simulink model "gcc"  (R2020a)
settings: Solver=ode23t  StartTime=0.0  StopTime=0.5  FixedStep=1e-6  RelTol=1e-3
undefined symbols (not defined in the file or in its folder): Ion, Lithium
libraries: powerlib x20, powerlib_extras x7, simulink x4, powerlib_meascontrol x2, electricdrivelib x1, re_lib x1
settings Model: Creator=kc  LastModifiedBy=BJ137
settings DataIOCC: SaveOutput=off  SignalLogging=off  DSMLogging=off  SaveTime=off  ReturnWorkspaceOutputs=off
settings OptimizationCC: LifeSpan=inf
settings DebuggingCC: ArithmeticOperatorsInVariantConditions=warning
settings SFSimCC: CustomCodeUndefinedFunction=UseInterfaceOnly
settings CodeAppCC: StateflowObjectComments=on

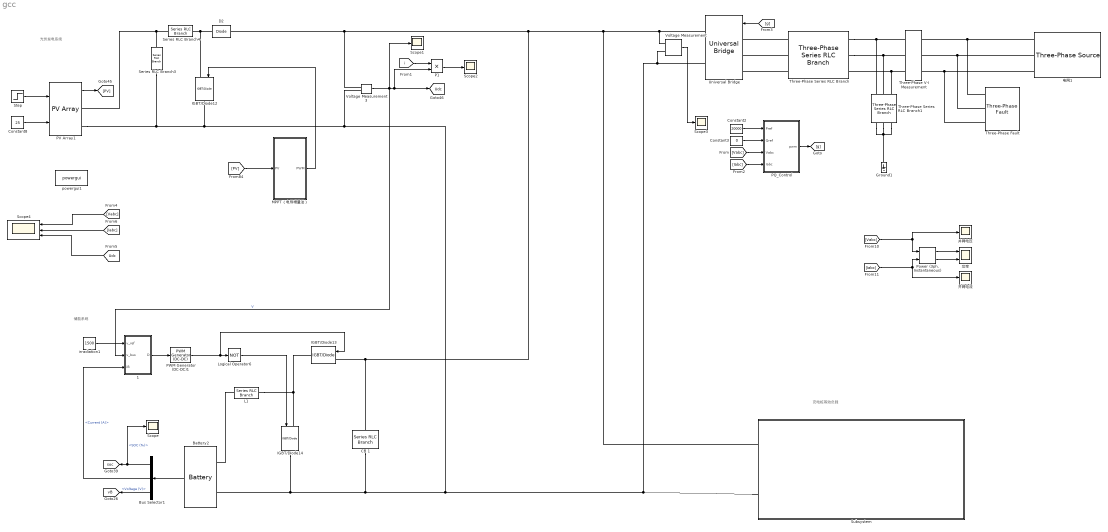
== system gcc ==
  note: 光伏发电系统
  note: 储能系统
  note: 充电桩等效负载
  1 : Subsystem
  Battery2 : electricdrivelib/Extra Sources/Battery  BatType=Lithium-Ion  ShowTempParam=off  ThermalPreset=no  ShowAgeParam=off  NomV=1000  NomQ=200  SOC=50  Batt_Tr=0  PresetModel=on  MaxQ=200  MinV=750  FullV=1163.9871  Dis_rate=86.9565  R=0.05  Normal_OP=180.8696  expZone="[1080.3859       9.826087]"  current=[6.5 13 32.5]  Units=Time  Tci=20  NomT=20  T2=-30  MaxQ2=4.8  FullV2=7.1  Normal_OP2=5.655  expZone2="[6.58           1]"  Rca=0.6  ti=2000  Dp=0  Neq0=0  Tsim=1e6  Ta1=25  Qeol=5.4*0.9  Reol=0.013333*1.2  Char_age=[2.3478, 3]  Dis_age=[2.3478, 10]  N1=1500  N2=10500  N3=1000  N4=1400  Ta2=45  N5=950
  Bus Selector1 : BusSelector  OutputSignals=SOC (%),Current (A),Voltage (V)
  CB 1 : powerlib/Elements/Series RLC Branch  LConnTagsString=__new0  RConnTagsString=__new0  BranchType=C  Resistance=1e-4  Inductance=1e-3  SetiL0=off  InitialCurrent=0  Capacitance=1000e-6  Setx0=on  InitialVoltage=800  Measurements=None
  Constant2 : Constant  Value=20000
  Constant3 : Constant  Value=0
  Constant8 : Constant  Value=25
  D2 : powerlib/Power Electronics/Diode  Ron=0.001  Lon=0  Vf=0  IC=0  UseSnubber=off  Rs=inf  Cs=inf  Measurements=off
  Ground1 : powerlib/Elements/Ground  LConnTagsString=a
  IGBT/Diode12 : powerlib/Power Electronics/IGBT//Diode  Ron=1e-3  Rs=1e5  Cs=inf  Measurements=off
  IGBT/Diode13 : powerlib/Power Electronics/IGBT//Diode  Ron=1e-3  Rs=1e5  Cs=inf  Measurements=off
  IGBT/Diode14 : powerlib/Power Electronics/IGBT//Diode  Ron=1e-3  Rs=1e5  Cs=inf  Measurements=off
  L1 : powerlib/Elements/Series RLC Branch  LConnTagsString=__new0  RConnTagsString=__new0  BranchType=RL  Resistance=0.1  Inductance=5e-3  SetiL0=off  InitialCurrent=0  Capacitance=100e-6  Setx0=off  InitialVoltage=0  Measurements=None
  Logical Operator6 : Logic  Operator=NOT  AllPortsSameDT=off  OutDataTypeStr=boolean
  MPPT （电导增量法） : Subsystem
  P1 : Product
  PQ_Control : Subsystem
  PV Array1 : re_lib/Solar/PV Array  Npar=660  Nser=12  PlotType=array @ 25 deg.C & specified irradiances  S_vec=[ 1000 ]  Temp_C_vec=[25]  ModuleName=China Sunergy (Nanjing) CSUN170-72M  PlotWhenSelected=off  Pm=170.016  Ncell=72  Voc=44.4  Isc=5.29  Vm=35.2  Im=4.83  beta_Voc_pc=-0.37563  alpha_Isc_pc=0.027391  beta_Voc=-0.16678  alpha_Isc=0.001449  IL=5.3113  I0=2.8712e-10  nI=1.0172  Rsh=192.6327  Rs=0.77439  RobustModel=off  RobustCellTemperature=313.3991  BAL=on  Tc=1e-6  Tfilter=50e-6
      settings: AttributesFormatString=|
      | %<ModuleName>
      | %<Nser>-module string
      | %<Npar> parallel strings
  PWM Generator (DC-DC)1 : powerlib_meascontrol/Pulse & Signal Generators/PWM Generator (DC-DC)  Fsw=5000  Ts=10e-6
  "Power (3ph, Instantaneous)" : powerlib_meascontrol/Measurements/Power (3ph, Instantaneous)
  Scope{,1..3} (4 alike) : Scope
  Scope4 : Scope  NumInputPorts=3
  Series RLC Branch3 : powerlib/Elements/Series RLC Branch  LConnTagsString=__new0  RConnTagsString=__new0  BranchType=C  Resistance=100e-3  Inductance=1e-3  SetiL0=off  InitialCurrent=0  Capacitance=100e-6  Setx0=off  InitialVoltage=0  Measurements=None
  Series RLC Branch4 : powerlib/Elements/Series RLC Branch  LConnTagsString=__new0  RConnTagsString=__new0  BranchType=L  Resistance=1  Inductance=0.6e-3  SetiL0=off  InitialCurrent=0  Capacitance=1e-6  Setx0=off  InitialVoltage=0  Measurements=None
  Step : Step  Time=0.3  Before=1000  After=1000  SampleTime=0
  Subsystem : Subsystem
  Three-Phase Series RLC Branch : powerlib/Elements/Three-Phase Series RLC Branch  LConnTagsString=A|B|C  RConnTagsString=A|B|C  BranchType=RL  Resistance=0.001  Inductance=9e-3  Capacitance=1e-6  Measurements=None
  Three-Phase Series RLC Branch1 : powerlib/Elements/Three-Phase Series RLC Branch  LConnTagsString=A|B|C  RConnTagsString=A|B|C  BranchType=RC  Resistance=0.01  Inductance=(2*pi*50*6e-3)/61.25  Capacitance=500e-6  Measurements=Branch voltages
  Three-Phase V-I Measurement : powerlib/Measurements/Three-Phase V-I Measurement  VoltageMeasurement=phase-to-ground  SetLabelV=on  LabelV=Vabc  Vpu=off  VpuLL=off  CurrentMeasurement=yes  SetLabelI=on  LabelI=Iabc  Ipu=off  Pbase=100e6  Vbase=500e3  OutputType=Complex  PhasorSimulation=off  PSBequivalent=0
  Three-Phase Fault : powerlib/Elements/Three-Phase Fault  InitialStates=0  FaultA=on  FaultB=on  FaultC=on  GroundFault=off  SwitchTimes=[0.3 0.35]  External=off  SwitchStatus=NaN  FaultResistance=0.01  GroundResistance=0.01  SnubberResistance=1e6  SnubberCapacitance=inf  Measurements=None
  Universal Bridge : powerlib/Power Electronics/Universal Bridge  Arms=3  SnubberResistance=1e5  SnubberCapacitance=inf  Device=IGBT / Diodes  Ron=1e-3  Lon=0  ForwardVoltages="[  0  0  ]"  ForwardVoltage=0  GTOparameters=[ 10e-6 , 20e-6 ]  IGBTparameters=[ 1e-6 , 2e-6 ]  Measurements=None  Measurements_2=None  converterType=Rectifier
  Voltage Measurement : powerlib/Measurements/Voltage Measurement  PhasorSimulation=off  OutputType=Complex  PSBequivalent=0
  Voltage Measurement3 : powerlib/Measurements/Voltage Measurement  PhasorSimulation=off  OutputType=Complex  PSBequivalent=0
  irradiation1 : Constant  Value=1500
  powergui1 : powerlib/powergui  Priority=1  SimulationMode=Discrete  SampleTime=1e-6  frequency=60  Iterations=50  frequencyindice=0  Pbase=100e6  ErrMax=1e-4  UnitsV=kV  UnitsW=MW  buscounter=0  FunctionMessages=off  echomessages=off  EnableUseOfTLC=off  CurrentSourceSwitches=off  DisableSnubberDevices=off  DisableRonSwitches=off  DisableVfSwitches=off  DisplayEquations=off  AutomaticDiscreteSolvers=off  SolverType=Tustin/Backward Euler (TBE)  Interpol=off  ExternalGateDelay=off  methode=off  Ts=100  x0status=blocks  SPID=on  SwTol=0  HookPort=off  NonlinearTolerance=1e-4  nMaxIteration=100  ContinueOnMaxIteration=off  RestoreLinks=warning  ResistiveCurrentMeasurement=off  Frange=[0:2:500]  Ylog=off  Xlog=on  ShowGrid=off  save=off  variable=ZData  structure=0  ZoomFFT=off  StartTime=0.0  cycles=1  DisplayStyle=1  fundamental=60  FreqAxis=off  MaxFrequency=1000  frequencyindicesteady=1  RmsSteady=1  display=off
  功率 : Scope  NumInputPorts=2
  并网电压 : Scope
  并网电流 : Scope
  电网1 : powerlib/Electrical Sources/Three-Phase Source  InternalConnection=Yg  VoltagePhases=off  Voltage=380  PhaseAngle=0  Voltage_phases=[25e3 25e3 25e3]/sqrt(3)  PhaseAngles_phases=[0 -120 +120]  Frequency=50  NonIdealSource=on  SpecifyImpedance=off  Resistance=0.1  Inductance=0  ShortCircuitLevel=100e6  BaseVoltage=25e3  XRratio=7  BusType=swing  Pref=0  Qref=0  Prefabc=[10e3, 10e3, 10e3]  Qrefabc=[0, 0, 0]  Qmin=-inf  Qmax=inf
  tag scope: Udc=global, soc=global, vB=global
  wires:
  Constant2/1 -> PQ_Control/1(Pref)
  Constant3/1 -> PQ_Control/2(Qref)
  [Iabc] -> "Power (3ph, Instantaneous)"/2, 并网电流/1
  "Power (3ph, Instantaneous)"/1 -> 功率/1
  [Vabc] -> "Power (3ph, Instantaneous)"/1, 并网电压/1
  "Power (3ph, Instantaneous)"/2 -> 功率/2
  [Vabc] -> PQ_Control/3(Vabc)
  [Iabc] -> PQ_Control/4(Iabc)
  PQ_Control/1(pwm) -> [g]
  [g] -> Universal Bridge/1
  Constant8/1 -> PV Array1/2
  [PV] -> MPPT （电导增量法）/1(PV)
  Voltage Measurement3/1 -> Scope1/1, P1/2, [Udc], 1/2(v_bus)  "V"
  Battery2/1 -> Bus Selector1/1
  1/1(D) -> PWM Generator (DC-DC)1/1
  PWM Generator (DC-DC)1/1 -> IGBT/Diode13/1, Logical Operator6/1
  Bus Selector1/3 -> [vB]  "<Voltage (V)>"
  PV Array1/1 -> [PV]
  irradiation1/1 -> 1/1(v_ref)
  Bus Selector1/1 -> Scope/1, [soc]  "<SOC (%)>"
  Step/1 -> PV Array1/1
  Logical Operator6/1 -> IGBT/Diode14/1
  Bus Selector1/2 -> 1/3(iB)  "<Current (A)>"
  [i] -> P1/1
  Voltage Measurement/1 -> Scope3/1
  P1/1 -> Scope2/1
  MPPT （电导增量法）/1(PWM) -> IGBT/Diode12/1
  [Vabc] -> Scope4/1
  [Udc] -> Scope4/3
  [Iabc] -> Scope4/2
  connections:
  Three-Phase V-I Measurement/LConn2 -- Three-Phase Series RLC Branch/RConn2 -- Three-Phase Series RLC Branch1/LConn2
  Three-Phase V-I Measurement/LConn3 -- Three-Phase Series RLC Branch/RConn3 -- Three-Phase Series RLC Branch1/LConn3
  Three-Phase V-I Measurement/LConn1 -- Three-Phase Series RLC Branch/RConn1 -- Three-Phase Series RLC Branch1/LConn1
  电网1/RConn2 -- Three-Phase Fault/LConn2 -- Three-Phase V-I Measurement/RConn2
  Three-Phase Series RLC Branch1/RConn1 -- Three-Phase Series RLC Branch1/RConn3 -- Ground1/LConn1 -- Three-Phase Series RLC Branch1/RConn2
  Three-Phase Series RLC Branch/LConn2 -- Universal Bridge/LConn2
  Three-Phase Series RLC Branch/LConn3 -- Universal Bridge/LConn3
  电网1/RConn1 -- Three-Phase Fault/LConn1 -- Three-Phase V-I Measurement/RConn1
  电网1/RConn3 -- Three-Phase Fault/LConn3 -- Three-Phase V-I Measurement/RConn3
  Series RLC Branch3/LConn1 -- PV Array1/RConn1 -- Series RLC Branch4/LConn1
  IGBT/Diode14/LConn1 -- L1/LConn1 -- IGBT/Diode13/RConn1
  IGBT/Diode12/LConn1 -- D2/LConn1 -- Series RLC Branch4/RConn1
  L1/RConn1 -- Battery2/LConn1
  CB 1/LConn1 -- Voltage Measurement/LConn1 -- Universal Bridge/RConn1 -- Subsystem/LConn1 -- D2/RConn1 -- Voltage Measurement3/LConn1 -- IGBT/Diode13/LConn1
  CB 1/RConn1 -- Battery2/LConn2 -- IGBT/Diode14/RConn1 -- Voltage Measurement3/LConn2 -- IGBT/Diode12/RConn1 -- Series RLC Branch3/RConn1 -- PV Array1/RConn2 -- Voltage Measurement/LConn2 -- Universal Bridge/RConn2 -- Subsystem/LConn2
  Three-Phase Series RLC Branch/LConn1 -- Universal Bridge/LConn1

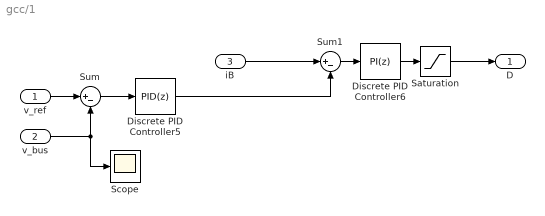
== system gcc/1 ==
  v_ref : Inport
  v_bus : Inport  Port=2
  iB : Inport  Port=3
  Discrete PID Controller5 : simulink/Continuous/PID Controller  Controller=PID  Form=Parallel  TimeDomain=Discrete-time  UseExternalTs=off  SampleTime=1e-6  IntegratorMethod=Forward Euler  FilterMethod=Forward Euler  ControllerParametersSource=internal  P=2  I=100  D=0  UseFilter=on  N=100  TunerSelectOption=Transfer Function Based (PID Tuner App)  InitialConditionSource=internal  InitialConditionForIntegrator=0  InitialConditionForFilter=0  DifferentiatorICPrevScaledInput=0  ExternalReset=none  TrackingMode=off  Kt=1  LimitOutput=on  UpperSaturationLimit=150  LowerSaturationLimit=-5000  LinearizeAsGain=off  AntiWindupMode=none  Kb=1  POutMin=[]  POutMax=[]  IOutMin=[]  IOutMax=[]  DOutMin=[]  DOutMax=[]  NOutMin=[]  NOutMax=[]  SumOutMin=[]  SumOutMax=[]  SaturationOutMin=[]  SaturationOutMax=[]  PParamMin=[]  PParamMax=[]  IParamMin=[]  IParamMax=[]  DParamMin=[]  DParamMax=[]  NParamMin=[]  NParamMax=[]  KbParamMin=[]  KbParamMax=[]  KtParamMin=[]  KtParamMax=[]  KbOutMin=[]  KbOutMax=[]  KtOutMin=[]  KtOutMax=[]  IntegratorOutMin=[]  IntegratorOutMax=[]  FilterOutMin=[]  FilterOutMax=[]  SumI1OutMin=[]  SumI1OutMax=[]  SumI2OutMin=[]  SumI2OutMax=[]  SumI3OutMin=[]  SumI3OutMax=[]  SumI4OutMin=[]  SumI4OutMax=[]  SumDOutMin=[]  SumDOutMax=[]  DifferentiatorOutMin=[]  DifferentiatorOutMax=[]  FilterDiffOutCoefMin=[]  FilterDiffOutCoefMax=[]  ReciprocalOutMin=[]  ReciprocalOutMax=[]  SumDenOutMin=[]  SumDenOutMax=[]  SumNumOutMin=[]  SumNumOutMax=[]  DivideOutMin=[]  DivideOutMax=[]  UdiffTsProdOutMin=[]  UdiffTsProdOutMax=[]  NTsProdOutMin=[]  NTsProdOutMax=[]  UintegralTsProdOutMin=[]  UintegralTsProdOutMax=[]  UngainTsProdOutMin=[]  UngainTsProdOutMax=[]  IntegratorContinuousStateAttributes=''  IntegratorStateMustResolveToSignalObject=off  IntegratorRTWStateStorageClass=Auto  FilterContinuousStateAttributes=''  FilterStateMustResolveToSignalObject=off  FilterRTWStateStorageClass=Auto  ParallelPVariant=InternalParameters  IdealPVariant=Disabled  IVariant=InternalParameters  DVariant=InternalParameters  IntegratorVariant=Discrete  SatVariant=Enabled  AWVariant=Passthrough  PCopyVariant=Disabled  TRVariant=Disabled  FdbkBlocksVariant=Forward  IdealPFdbkVariant=Disabled  SatFdbkVariant=Disabled  DerivativeFilterVariant=ForwardEulerFilter  NVariant=InternalParameters  NCopyVariant=Disabled  FilterICVariant=InternalICsFilter  IntegratorICVariant=InternalICs  ExternalResetVariant=Disabled  TRSumVariant=Passthrough  SumFdbkVariant=Disabled  SumVariant=Sum_PID  TsampFilterVariant=InternalTs  TsampNgainVariant=Passthrough  TsampIntegralVariant=Passthrough
  Discrete PID Controller6 : simulink/Continuous/PID Controller  Controller=PI  Form=Parallel  TimeDomain=Discrete-time  UseExternalTs=off  SampleTime=50e-6  IntegratorMethod=Forward Euler  FilterMethod=Forward Euler  ControllerParametersSource=internal  P=0.02  I=10  D=0  UseFilter=on  N=100  TunerSelectOption=Transfer Function Based (PID Tuner App)  InitialConditionSource=internal  InitialConditionForIntegrator=0  InitialConditionForFilter=0  DifferentiatorICPrevScaledInput=0  ExternalReset=none  TrackingMode=off  Kt=1  LimitOutput=off  UpperSaturationLimit=0.9  LowerSaturationLimit=0.1  LinearizeAsGain=off  AntiWindupMode=none  Kb=1  POutMin=[]  POutMax=[]  IOutMin=[]  IOutMax=[]  DOutMin=[]  DOutMax=[]  NOutMin=[]  NOutMax=[]  SumOutMin=[]  SumOutMax=[]  SaturationOutMin=[]  SaturationOutMax=[]  PParamMin=[]  PParamMax=[]  IParamMin=[]  IParamMax=[]  DParamMin=[]  DParamMax=[]  NParamMin=[]  NParamMax=[]  KbParamMin=[]  KbParamMax=[]  KtParamMin=[]  KtParamMax=[]  KbOutMin=[]  KbOutMax=[]  KtOutMin=[]  KtOutMax=[]  IntegratorOutMin=[]  IntegratorOutMax=[]  FilterOutMin=[]  FilterOutMax=[]  SumI1OutMin=[]  SumI1OutMax=[]  SumI2OutMin=[]  SumI2OutMax=[]  SumI3OutMin=[]  SumI3OutMax=[]  SumI4OutMin=[]  SumI4OutMax=[]  SumDOutMin=[]  SumDOutMax=[]  DifferentiatorOutMin=[]  DifferentiatorOutMax=[]  FilterDiffOutCoefMin=[]  FilterDiffOutCoefMax=[]  ReciprocalOutMin=[]  ReciprocalOutMax=[]  SumDenOutMin=[]  SumDenOutMax=[]  SumNumOutMin=[]  SumNumOutMax=[]  DivideOutMin=[]  DivideOutMax=[]  UdiffTsProdOutMin=[]  UdiffTsProdOutMax=[]  NTsProdOutMin=[]  NTsProdOutMax=[]  UintegralTsProdOutMin=[]  UintegralTsProdOutMax=[]  UngainTsProdOutMin=[]  UngainTsProdOutMax=[]  IntegratorContinuousStateAttributes=''  IntegratorStateMustResolveToSignalObject=off  IntegratorRTWStateStorageClass=Auto  FilterContinuousStateAttributes=''  FilterStateMustResolveToSignalObject=off  FilterRTWStateStorageClass=Auto  ParallelPVariant=InternalParameters  IdealPVariant=Disabled  IVariant=InternalParameters  DVariant=Disabled  IntegratorVariant=Discrete  SatVariant=Disabled  AWVariant=Passthrough  PCopyVariant=Disabled  TRVariant=Disabled  FdbkBlocksVariant=Forward  IdealPFdbkVariant=Disabled  SatFdbkVariant=Disabled  DerivativeFilterVariant=Disabled  NVariant=Disabled  NCopyVariant=Disabled_SignalSpec  FilterICVariant=Disabled  IntegratorICVariant=InternalICs  ExternalResetVariant=Disabled  TRSumVariant=Passthrough  SumFdbkVariant=Disabled  SumVariant=Sum_PI  TsampFilterVariant=InternalTs  TsampNgainVariant=Passthrough  TsampIntegralVariant=Passthrough
  Saturation : Saturate  UpperLimit=0.9  LowerLimit=0.1
  Scope : Scope
  Sum : Sum  Inputs=|+-
  Sum1 : Sum  Inputs=|+-
  D : Outport
  wires:
  v_ref/1 -> Sum/1
  Sum1/1 -> Discrete PID Controller6/1
  Discrete PID Controller6/1 -> Saturation/1
  iB/1 -> Sum1/1
  v_bus/1 -> Scope/1, Sum/2
  Discrete PID Controller5/1 -> Sum1/2
  Sum/1 -> Discrete PID Controller5/1
  Saturation/1 -> D/1

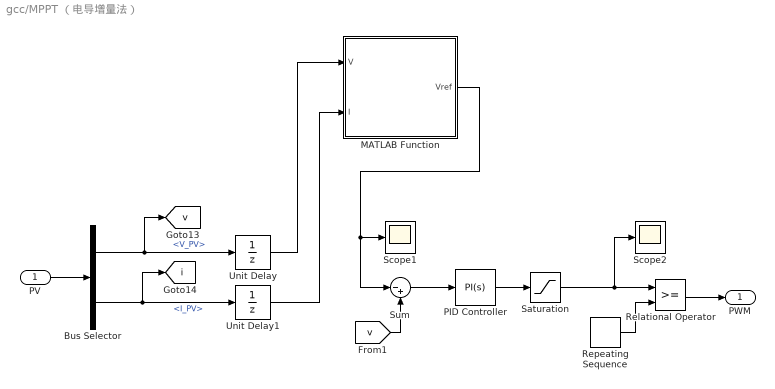
== system gcc/MPPT （电导增量法） ==
  PV : Inport
  Bus Selector : BusSelector  OutputSignals=V_PV,I_PV
  MATLAB Function : MATLAB Function  TreatAsAtomicUnit=on
  PID Controller : simulink/Continuous/PID Controller  Controller=PI  Form=Parallel  TimeDomain=Continuous-time  UseExternalTs=off  SampleTime=-1  IntegratorMethod=Forward Euler  FilterMethod=Forward Euler  ControllerParametersSource=internal  P=0.0025  I=0.58  D=0  UseFilter=on  N=100  TunerSelectOption=Transfer Function Based (PID Tuner App)  InitialConditionSource=internal  InitialConditionForIntegrator=0  InitialConditionForFilter=0  DifferentiatorICPrevScaledInput=0  ExternalReset=none  TrackingMode=off  Kt=1  LimitOutput=off  UpperSaturationLimit=1  LowerSaturationLimit=0  LinearizeAsGain=on  AntiWindupMode=none  Kb=1  POutMin=[]  POutMax=[]  IOutMin=[]  IOutMax=[]  DOutMin=[]  DOutMax=[]  NOutMin=[]  NOutMax=[]  SumOutMin=[]  SumOutMax=[]  SaturationOutMin=[]  SaturationOutMax=[]  PParamMin=[]  PParamMax=[]  IParamMin=[]  IParamMax=[]  DParamMin=[]  DParamMax=[]  NParamMin=[]  NParamMax=[]  KbParamMin=[]  KbParamMax=[]  KtParamMin=[]  KtParamMax=[]  KbOutMin=[]  KbOutMax=[]  KtOutMin=[]  KtOutMax=[]  IntegratorOutMin=[]  IntegratorOutMax=[]  FilterOutMin=[]  FilterOutMax=[]  SumI1OutMin=[]  SumI1OutMax=[]  SumI2OutMin=[]  SumI2OutMax=[]  SumI3OutMin=[]  SumI3OutMax=[]  SumI4OutMin=[]  SumI4OutMax=[]  SumDOutMin=[]  SumDOutMax=[]  DifferentiatorOutMin=[]  DifferentiatorOutMax=[]  FilterDiffOutCoefMin=[]  FilterDiffOutCoefMax=[]  ReciprocalOutMin=[]  ReciprocalOutMax=[]  SumDenOutMin=[]  SumDenOutMax=[]  SumNumOutMin=[]  SumNumOutMax=[]  DivideOutMin=[]  DivideOutMax=[]  UdiffTsProdOutMin=[]  UdiffTsProdOutMax=[]  NTsProdOutMin=[]  NTsProdOutMax=[]  UintegralTsProdOutMin=[]  UintegralTsProdOutMax=[]  UngainTsProdOutMin=[]  UngainTsProdOutMax=[]  IntegratorContinuousStateAttributes=''  IntegratorStateMustResolveToSignalObject=off  IntegratorRTWStateStorageClass=Auto  FilterContinuousStateAttributes=''  FilterStateMustResolveToSignalObject=off  FilterRTWStateStorageClass=Auto  ParallelPVariant=InternalParameters  IdealPVariant=Disabled  IVariant=InternalParameters  DVariant=Disabled  IntegratorVariant=Continuous  SatVariant=Disabled  AWVariant=Passthrough  PCopyVariant=Disabled  TRVariant=Disabled  FdbkBlocksVariant=Forward  IdealPFdbkVariant=Disabled  SatFdbkVariant=Disabled  DerivativeFilterVariant=Disabled  NVariant=Disabled  NCopyVariant=Disabled_SignalSpec  FilterICVariant=Disabled  IntegratorICVariant=InternalICs  ExternalResetVariant=Disabled  TRSumVariant=Passthrough  SumFdbkVariant=Disabled  SumVariant=Sum_PI  TsampFilterVariant=InternalTs  TsampNgainVariant=Passthrough  TsampIntegralVariant=Passthrough
  Relational Operator : RelationalOperator  OutDataTypeStr=boolean  RndMeth=Nearest
  Repeating Sequence : simulink/Sources/Repeating Sequence  rep_seq_t=[0 1/20000]  rep_seq_y=[0 1]
  Saturation : Saturate  UpperLimit=1  LowerLimit=0
  Scope1 : Scope
  Scope2 : Scope
  Sum : Sum  Inputs=|-+
  Unit Delay : UnitDelay  SampleTime=1/10000  HasFrameUpgradeWarning=on
  Unit Delay1 : UnitDelay  SampleTime=1/10000  HasFrameUpgradeWarning=on
  PWM : Outport
  tag scope: i=global, v=global
  wires:
  MATLAB Function/1(Vref) -> Sum/1, Scope1/1
  Repeating Sequence/1 -> Relational Operator/2
  PID Controller/1 -> Saturation/1
  Sum/1 -> PID Controller/1
  Unit Delay1/1 -> MATLAB Function/2(I)
  Unit Delay/1 -> MATLAB Function/1(V)
  Bus Selector/1 -> [v], Unit Delay/1  "<V_PV>"
  Bus Selector/2 -> [i], Unit Delay1/1  "<I_PV>"
  PV/1 -> Bus Selector/1
  Relational Operator/1 -> PWM/1
  [v] -> Sum/2
  Saturation/1 -> Relational Operator/1, Scope2/1

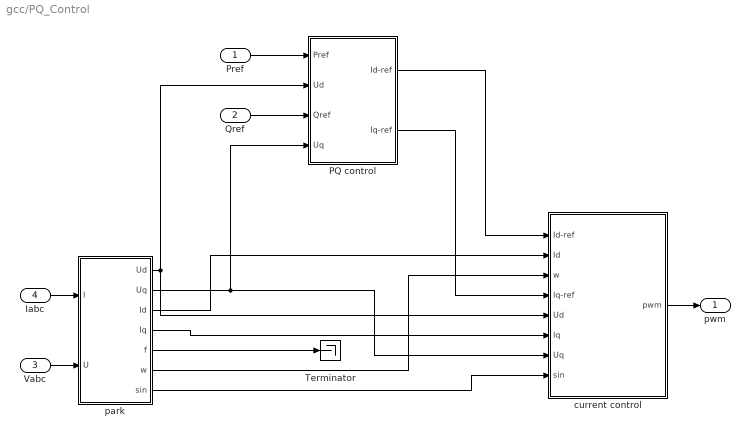
== system gcc/PQ_Control ==
  Pref : Inport
  Qref : Inport  Port=2
  Vabc : Inport  Port=3
  Iabc : Inport  Port=4
  PQ control : Subsystem
  Terminator : Terminator
  current control : Subsystem
  park : Subsystem
  pwm : Outport
  wires:
  Iabc/1 -> park/1(I)
  Vabc/1 -> park/2(U)
  Pref/1 -> PQ control/1(Pref)
  current control/1(pwm) -> pwm/1
  park/7(sin) -> current control/8(sin)
  park/6(w) -> current control/3(w)
  park/4(Iq) -> current control/6(Iq)
  park/3(Id) -> current control/2(Id)
  park/2(Uq) -> current control/7(Uq), PQ control/4(Uq)
  PQ control/2(Iq-ref) -> current control/4(Iq-ref)
  PQ control/1(Id-ref) -> current control/1(Id-ref)
  park/5(f) -> Terminator/1
  Qref/1 -> PQ control/3(Qref)
  park/1(Ud) -> PQ control/2(Ud), current control/5(Ud)

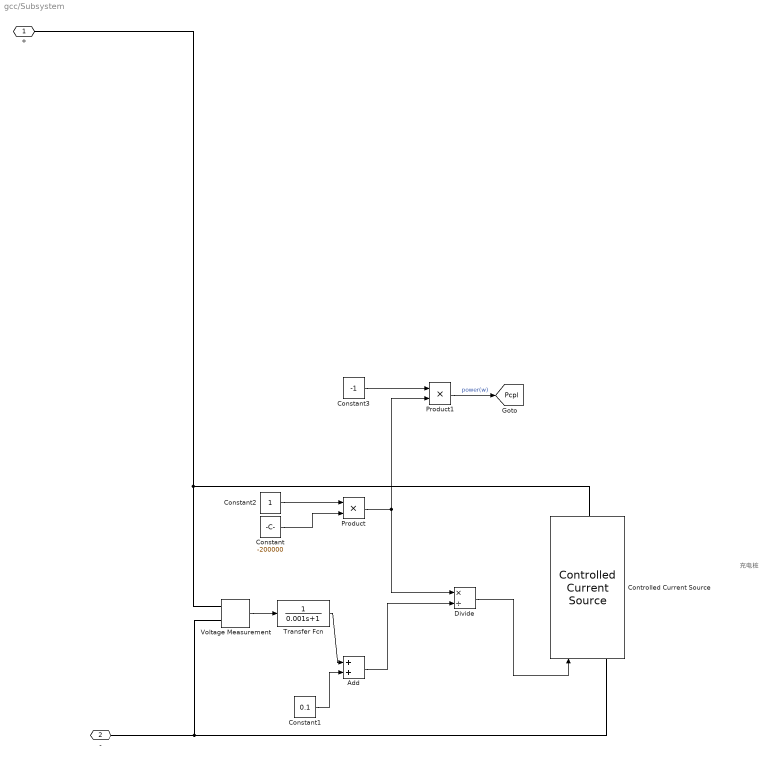
== system gcc/Subsystem ==
  note: 充电桩
  Add : Sum
  Constant : Constant  Value=-200000
  Constant1 : Constant  Value=0.1
  Constant2 : Constant
  Constant3 : Constant  Value=-1
  Controlled Current Source : powerlib/Electrical Sources/Controlled Current Source  Initialize=on  Source_Type=DC  Amplitude=0  Phase=0  Frequency=0  Measurements=None
  Divide : Product  Inputs=*/
  Product : Product
  Product1 : Product
  Transfer Fcn : TransferFcn  Denominator=[0.001 1]
  Voltage Measurement : powerlib/Measurements/Voltage Measurement  PhasorSimulation=off  OutputType=Complex  PSBequivalent=0
  + : PMIOPort  Side=Left
  - : PMIOPort  Port=2  Side=Left
  tag scope: Pcpl=global
  wires:
  Add/1 -> Divide/2
  Transfer Fcn/1 -> Add/1
  Product/1 -> Product1/2, Divide/1
  Constant/1 -> Product/2
  Divide/1 -> Controlled Current Source/1
  Constant1/1 -> Add/2
  Voltage Measurement/1 -> Transfer Fcn/1
  Product1/1 -> [Pcpl]  "power(w)"
  Constant3/1 -> Product1/1
  Constant2/1 -> Product/1
  connections:
  Controlled Current Source/RConn1 -- +/RConn1 -- Voltage Measurement/LConn1
  Controlled Current Source/LConn1 -- -/RConn1 -- Voltage Measurement/LConn2

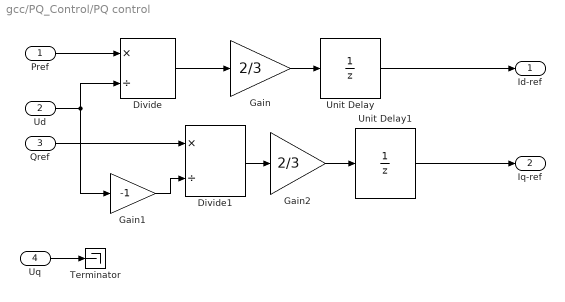
== system gcc/PQ_Control/PQ control ==
  Pref : Inport
  Ud : Inport  Port=2
  Qref : Inport  Port=3
  Uq : Inport  Port=4
  Divide : Product  Inputs=*/
  Divide1 : Product  Inputs=*/
  Gain : Gain  Gain=2/3
  Gain1 : Gain  Gain=-1
  Gain2 : Gain  Gain=2/3
  Terminator : Terminator
  Unit Delay : UnitDelay  SampleTime=-1  HasFrameUpgradeWarning=on
  Unit Delay1 : UnitDelay  SampleTime=-1  HasFrameUpgradeWarning=on
  Id-ref : Outport
  Iq-ref : Outport  Port=2
  wires:
  Uq/1 -> Terminator/1
  Pref/1 -> Divide/1
  Ud/1 -> Divide/2, Gain1/1
  Gain1/1 -> Divide1/2
  Unit Delay1/1 -> Iq-ref/1
  Qref/1 -> Divide1/1
  Unit Delay/1 -> Id-ref/1
  Divide/1 -> Gain/1
  Gain/1 -> Unit Delay/1
  Divide1/1 -> Gain2/1
  Gain2/1 -> Unit Delay1/1

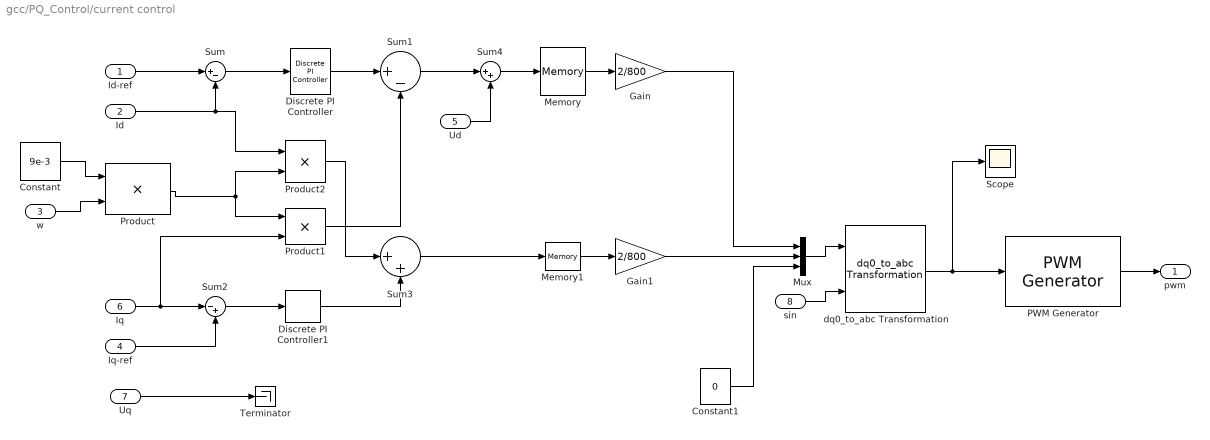
== system gcc/PQ_Control/current control ==
  Id-ref : Inport
  Id : Inport  Port=2
  w : Inport  Port=3
  Iq-ref : Inport  Port=4
  Ud : Inport  Port=5
  Iq : Inport  Port=6
  Uq : Inport  Port=7
  sin : Inport  Port=8
  Constant : Constant  Value=9e-3
  Constant1 : Constant  Value=0
  Discrete PI Controller : powerlib_extras/Discrete  Control Blocks/Discrete PI Controller  Kp=20  Ki=250  Par_Limits=[1e6 -1e6]  Init=0  Ts=50e-6
  Discrete PI Controller1 : powerlib_extras/Discrete  Control Blocks/Discrete PI Controller  Kp=20  Ki=250  Par_Limits=[1e6 -1e6]  Init=0  Ts=50e-6
  Gain : Gain  Gain=2/800
  Gain1 : Gain  Gain=2/800
  Memory : Memory
  Memory1 : Memory
  Mux : Mux  Inputs=3
  PWM Generator : powerlib_extras/Control  Blocks/PWM Generator  GeneratorMode="3-arm  bridge (6 pulses)"  Fc=8000  Internal=off  mIndex=0.4  Freq=60  Phase=0
      settings: SourceProductBaseCode=PS
  Product : Product  RndMeth=Zero
  Product1 : Product  RndMeth=Zero
  Product2 : Product  RndMeth=Zero
  Scope : Scope
  Sum : Sum  Inputs=|+-
  Sum1 : Sum  Inputs=|+-
  Sum2 : Sum  Inputs=|-+
  Sum3 : Sum  Inputs=|++
  Sum4 : Sum  Inputs=|++
  Terminator : Terminator
  dq0_to_abc Transformation : powerlib_extras/Measurements/dq0_to_abc Transformation
      settings: SourceProductBaseCode=PS
  pwm : Outport
  wires:
  Id-ref/1 -> Sum/1
  Id/1 -> Sum/2, Product2/1
  Sum/1 -> Discrete PI Controller/1
  Discrete PI Controller/1 -> Sum1/1
  Constant/1 -> Product/1
  w/1 -> Product/2
  Product/1 -> Product1/1, Product2/2
  Product1/1 -> Sum1/2
  Iq/1 -> Sum2/1, Product1/2
  Iq-ref/1 -> Sum2/2
  Sum2/1 -> Discrete PI Controller1/1
  Product2/1 -> Sum3/1
  Discrete PI Controller1/1 -> Sum3/2
  Uq/1 -> Terminator/1
  Sum1/1 -> Sum4/1
  Ud/1 -> Sum4/2
  Constant1/1 -> Mux/3
  Mux/1 -> dq0_to_abc Transformation/1
  sin/1 -> dq0_to_abc Transformation/2
  dq0_to_abc Transformation/1 -> Scope/1, PWM Generator/1
  PWM Generator/1 -> pwm/1
  Sum4/1 -> Memory/1
  Sum3/1 -> Memory1/1
  Memory/1 -> Gain/1
  Gain/1 -> Mux/1
  Memory1/1 -> Gain1/1
  Gain1/1 -> Mux/2

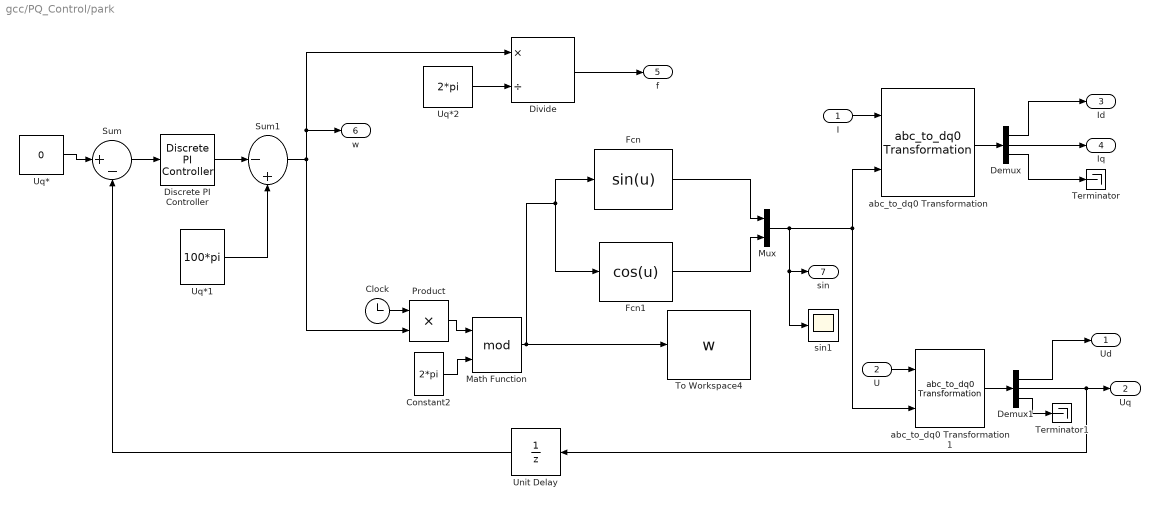
== system gcc/PQ_Control/park ==
  I : Inport
  U : Inport  Port=2
  Clock : Clock
  Constant2 : Constant  Value=2*pi
  Demux : Demux  Outputs=3
  Demux1 : Demux  Outputs=3
  Discrete PI Controller : powerlib_extras/Discrete  Control Blocks/Discrete PI Controller  Kp=0.0007  Ki=0.833  Par_Limits=[1e6 -1e6]  Init=0  Ts=50e-6
  Divide : Product  Inputs=*/
  Fcn : Fcn  Expr=sin(u)
  Fcn1 : Fcn  Expr=cos(u)
  Math Function : Math  Operator=mod  SignedPower=on  SaturateOnIntegerOverflow=on
  Mux : Mux  Inputs=2
  Product : Product  RndMeth=Zero
  Sum : Sum  Inputs=|+-
  Sum1 : Sum  Inputs=|-+
  Terminator : Terminator
  Terminator1 : Terminator
  To Workspace4 : ToWorkspace  VariableName=w  SaveFormat=Timeseries  SampleTime=-1
  Unit Delay : UnitDelay  SampleTime=-1  HasFrameUpgradeWarning=on
  Uq* : Constant  Value=0
  Uq*1 : Constant  Value=100*pi
  Uq*2 : Constant  Value=2*pi
  abc_to_dq0 Transformation : powerlib_extras/Measurements/abc_to_dq0 Transformation
      settings: SourceProductBaseCode=PS
  abc_to_dq0 Transformation1 : powerlib_extras/Measurements/abc_to_dq0 Transformation
      settings: SourceProductBaseCode=PS
  sin1 : Scope
  Ud : Outport
  Uq : Outport  Port=2
  Id : Outport  Port=3
  Iq : Outport  Port=4
  f : Outport  Port=5
  w : Outport  Port=6
  sin : Outport  Port=7
  wires:
  Demux1/3 -> Terminator1/1
  Demux1/2 -> Uq/1, Unit Delay/1
  Demux1/1 -> Ud/1
  abc_to_dq0 Transformation1/1 -> Demux1/1
  U/1 -> abc_to_dq0 Transformation1/1
  Demux/2 -> Iq/1
  Demux/1 -> Id/1
  Demux/3 -> Terminator/1
  abc_to_dq0 Transformation/1 -> Demux/1
  I/1 -> abc_to_dq0 Transformation/1
  Sum1/1 -> Product/2, Divide/1, w/1
  Product/1 -> Math Function/1
  Divide/1 -> f/1
  Mux/1 -> abc_to_dq0 Transformation/2, abc_to_dq0 Transformation1/2, sin/1, sin1/1
  Fcn1/1 -> Mux/2
  Fcn/1 -> Mux/1
  Math Function/1 -> To Workspace4/1, Fcn/1, Fcn1/1
  Constant2/1 -> Math Function/2
  Uq*2/1 -> Divide/2
  Clock/1 -> Product/1
  Uq*1/1 -> Sum1/2
  Discrete PI Controller/1 -> Sum1/1
  Sum/1 -> Discrete PI Controller/1
  Uq*/1 -> Sum/1
  Unit Delay/1 -> Sum/2

== matlab function gcc/MPPT （电导增量法）/MATLAB Function ==
  data: V input; Vref output; I input
 function Vref= fcn(V,I)
Vrefmax=444;
Vrefmin=0;
Vref_init=352;
delta_Vref=0.001;  %步长

persistent Vold Iold Vrefold; %其值保留在对该函数的多次调用所使用的内存中

%dataType = 'double'; %初始赋值
if isempty(Vold)
    Vold=0;
    Iold=0;
    Vrefold=Vref_init;
end

dV= V - Vold;
dI= I - Iold;
X=dI/dV;
Y=-I/V;

if dV  ~= 0 
    if X ~= Y
        if X > Y
            Vref= Vrefold + delta_Vref;
        else
            Vref= Vrefold - delta_Vref;
        end
    else
        Vref= Vrefold;
    end
else
        if dI ~= 0 
            if dI > 0 
            Vref= Vrefold + delta_Vref;
        else
            Vref= Vrefold - delta_Vref;
            end 
        else
             Vref= Vrefold;
        end
end

if Vref>= Vrefmax||Vref<= Vrefmin
   Vref=Vrefold;
end  

Vrefold=Vref;
Vold=V;
Iold=I;
end
